simulink model "single_phase_PWM_inverter"  (R2024b)
settings: Solver=VariableStepAuto  StartTime=0.0  StopTime=1  RelTol=1e-3
libraries: spsMosfetLib x4, spsMultimeterLib x2, spsDCVoltageSourceLib x1, spsFourierLib x1, spsMeanLib x1, spsRMSLib x1, simulink x1, spsSeriesRLCBranchLib x1, sps_lib x1
settings Model: Creator=User  LastModifiedBy=User

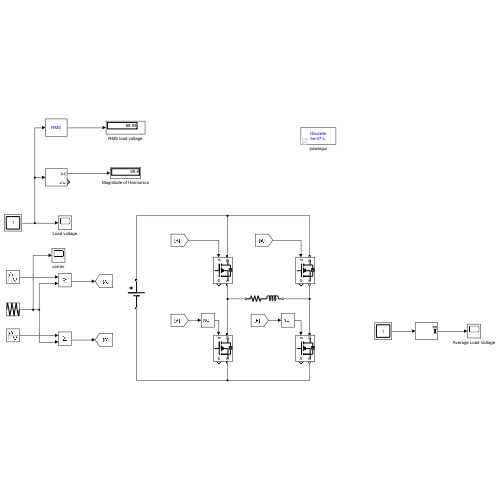
[thumbnail: Simulink's stored preview of the top-level diagram]
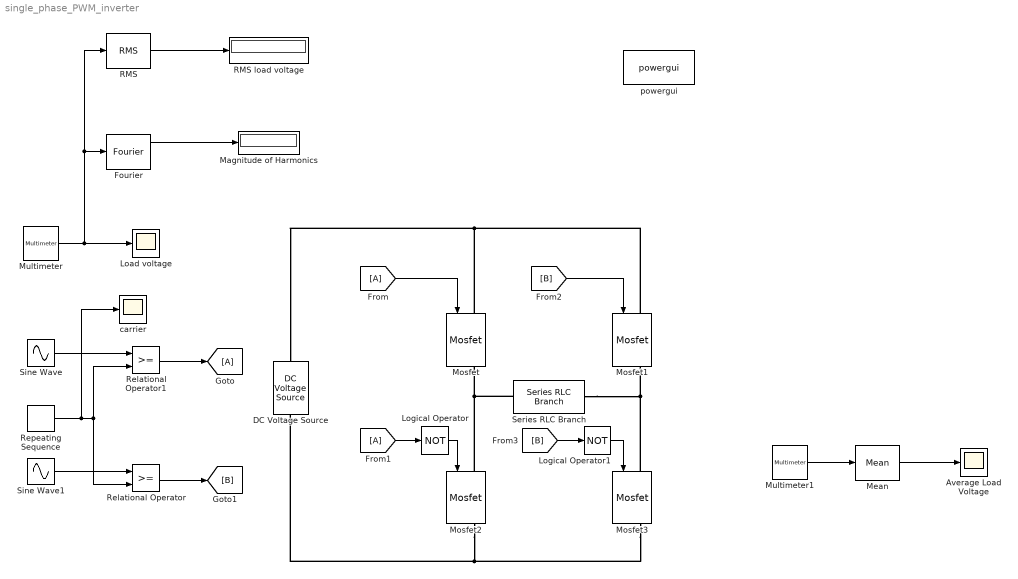
== system single_phase_PWM_inverter ==
  Average Load Voltage : Scope
  DC Voltage Source : spsDCVoltageSourceLib/DC Voltage Source  Amplitude=100  Measurements=None
  Fourier : spsFourierLib/Fourier  Freq=60  n=1  InInit=[0, 0]  Ts=0
  From : From
  From1 : From
  Goto : Goto
  Load voltage : Scope
  Logical Operator : Logic  Operator=NOT  AllPortsSameDT=off  OutDataTypeStr=boolean
  Logical Operator1 : Logic  Operator=NOT  AllPortsSameDT=off  OutDataTypeStr=boolean
  Magnitude of Harmonics : Display
  Mean : spsMeanLib/Mean  Freq=23*50  Vinit=0  Ts=0
  Mosfet{,1..3} (4 alike) : spsMosfetLib/Mosfet  Ron=0.1  Lon=0  Rd=0.01  Vfd=0  IC=0  Rs=1e5  Cs=inf  Measurements=on
  Multimeter : spsMultimeterLib/Multimeter  L=1  sel=1  yselected={}  Gain=1  OutputType=Complex  PlotAtSimulationStop=off  PhasorSimulation=off
  Multimeter1 : spsMultimeterLib/Multimeter  L=1  sel=1  yselected={}  Gain=1  OutputType=Complex  PlotAtSimulationStop=off  PhasorSimulation=off
  RMS : spsRMSLib/RMS  TrueRMS=on  Freq=60  RMSInit=120  Ts=0
  RMS load voltage : Display
  Relational Operator : RelationalOperator  OutDataTypeStr=boolean  RndMeth=Simplest  InputSameDT=off
  Relational Operator1 : RelationalOperator  OutDataTypeStr=boolean  RndMeth=Simplest  InputSameDT=off
  Repeating Sequence : simulink/Sources/Repeating Sequence  rep_seq_t=[0 1 2 3 4]*1/(23*50*4)  rep_seq_y=[0 1 0 -1 0]
  Series RLC Branch : spsSeriesRLCBranchLib/Series RLC Branch  LConnTagsString=__new0  RConnTagsString=__new0  BranchType=RL  Resistance=25  Inductance=1e-3  SetiL0=off  InitialCurrent=0  Capacitance=1e-6  Setx0=off  InitialVoltage=0  Measurements=Branch voltage
  Sine Wave : Sin  Amplitude=0.7  Frequency=2*pi*50  SampleTime=0
  Sine Wave1 : Sin  Amplitude=0.7  Frequency=2*pi*50  Phase=pi  SampleTime=0
  carrier : Scope
  powergui : sps_lib/powergui  Priority=1  SimulationMode=Discrete  SampleTime=5e-7  frequency=60  Iterations=50  frequencyindice=0  Pbase=100e6  ErrMax=1e-4  UnitsV=kV  UnitsW=MW  buscounter=0  FunctionMessages=off  echomessages=off  EnableUseOfTLC=off  CurrentSourceSwitches=off  DisableSnubberDevices=off  DisableRonSwitches=off  DisableVfSwitches=off  DisplayEquations=off  AutomaticDiscreteSolvers=off  SolverType=Tustin/Backward Euler (TBE)  Interpol=off  ExternalGateDelay=off  methode=off  Ts=100  x0status=blocks  SPID=on  SwTol=0  HookPort=off  NonlinearTolerance=1e-4  nMaxIteration=100  ContinueOnMaxIteration=off  RestoreLinks=warning  ResistiveCurrentMeasurement=off  Frange=[0:2:500]  Ylog=off  Xlog=on  ShowGrid=off  save=off  variable=ZData  structure=0  ZoomFFT=off  StartTime=0.0  cycles=1  DisplayStyle=1  fundamental=60  FreqAxis=off  MaxFrequency=1000  frequencyindicesteady=1  RmsSteady=1  display=off
  wires:
  From/1 -> Mosfet/1
  From1/1 -> Logical Operator/1
  Logical Operator/1 -> Mosfet2/1
  [B] -> Mosfet1/1
  [B] -> Logical Operator1/1
  Logical Operator1/1 -> Mosfet3/1
  Multimeter/1 -> Fourier/1, RMS/1, Load voltage/1
  Relational Operator1/1 -> Goto/1
  Relational Operator/1 -> [B]
  Sine Wave/1 -> Relational Operator1/1
  Repeating Sequence/1 -> carrier/1, Relational Operator/2, Relational Operator1/2
  Sine Wave1/1 -> Relational Operator/1
  Multimeter1/1 -> Mean/1
  Mean/1 -> Average Load Voltage/1
  RMS/1 -> RMS load voltage/1
  Fourier/1 -> Magnitude of Harmonics/1
  connections:
  Series RLC Branch/RConn1 -- Mosfet1/RConn1 -- Mosfet3/LConn1
  Mosfet2/LConn1 -- Series RLC Branch/LConn1 -- Mosfet/RConn1
  Mosfet/LConn1 -- Mosfet1/LConn1 -- DC Voltage Source/RConn1
  Mosfet2/RConn1 -- Mosfet3/RConn1 -- DC Voltage Source/LConn1
